simulink model "simulinkGit"  (R2024b)
settings: Solver=FixedStepDiscrete  StartTime=0.0  StopTime=10.0  RelTol=1e-3
model workspace (MAT data in the model file):
  firstWarning = 1
  originalScenarioChecksum = 'CA9770AAA36CFFEF06F2135ABF4DE208'
undefined symbols (not defined in the file or in its folder): driving
libraries: drivingscenarioandsensors x5, sensorinslib x1
(part 1 of 2)
settings Model: Creator=1111a  LastModifiedBy=1111a

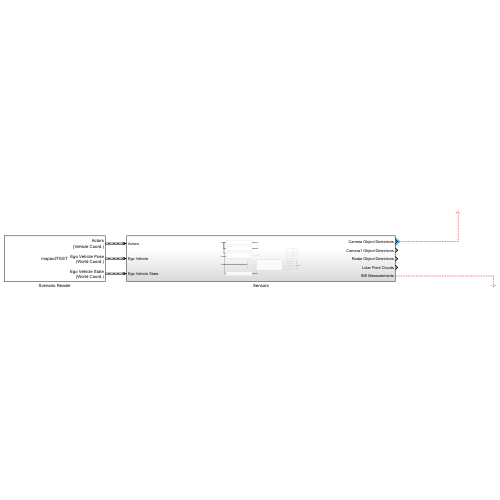
[thumbnail: Simulink's stored preview of the top-level diagram]
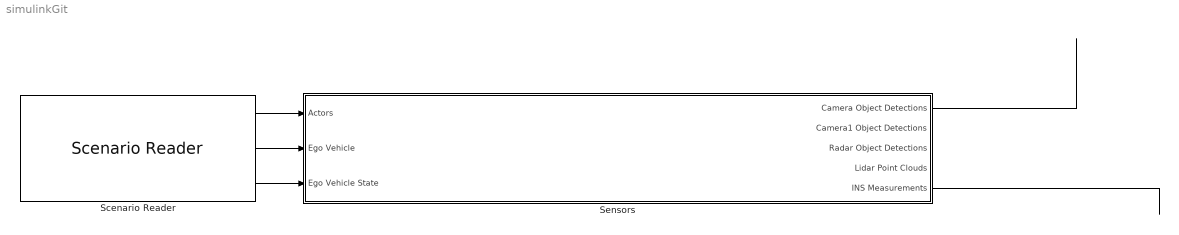
== system simulinkGit ==
  Scenario Reader : drivingscenarioandsensors/Scenario Reader  ScenarioSource=From file  ScenarioFileName=C:\Users\1111a\Desktop\Studia\ms\MISSwR-Laby\MISSwR-Laby\lab2\mapav2TEST.mat  ScenarioVariableName=scenario  OutputCoordinateSystem=Vehicle coordinates  EgoVehicleSource=Scenario  EgoVehicleActorID=1  OrientVehiclesOnRoad=off  OutputEgoVehiclePose=on  OutputEgoVehicleState=on  SampleTime=0.1  LaneBoundaryOutput=None  LaneBoundaryDistance=0:0.5:9.5  LaneBoundaryLocation=Center of lane markings  BusNameSource=Auto  BusName=BusActors  BusNumActorsSource=Scenario  BusNumActors=100  BusName2Source=Auto  BusName2=BusLaneBoundaries  BusNumLaneBoundariesSource=Scenario  BusNumLaneBoundaries=10  BusName3Source=Auto  BusName3=BusEgoActor  BusName4Source=Auto  BusName4=BusEgoState  ShowCoordinateLabels=on  SimulateUsing=Interpreted execution
  Sensors : Subsystem
  wires:
  Scenario Reader/3 -> Sensors/3(Ego Vehicle State)
  Scenario Reader/2 -> Sensors/2(Ego Vehicle)
  Scenario Reader/1 -> Sensors/1(Actors)
  Sensors/5(INS Measurements) -> ?
  Sensors/1(Camera Object Detections) -> ?
